simulink model "BS_Adaptive"  (R2018b)
settings: Solver=VariableStepAuto  StartTime=0.0  StopTime=10  RelTol=1e-3
values from neighbouring files (symbols this model uses):
  cond_init = [0, 150/180*pi, pi/3, -pi/2, -3*pi/4,-150/180*pi]'    [init.m]
  hand_des = p(6,:)'    [init.m]
  Law_param = [kd,kd,kd,kd,kd,kd ... (first row only)    [LAUNCH_Backstepping.m]    (also in LAUNCH_Backstepping_Adaptavive.m = [kp,kp,kp,kp,kp,kp; LAUNCH_PD_TRAJ.m = [300000,300000,300000,300000,300000,300000)
  param = param'    [init.m]
  pi_0 = 1    [LAUNCH_Backstepping_Adaptavive.m]
settings Model: Creator=Utente  LastModifiedBy=Utente

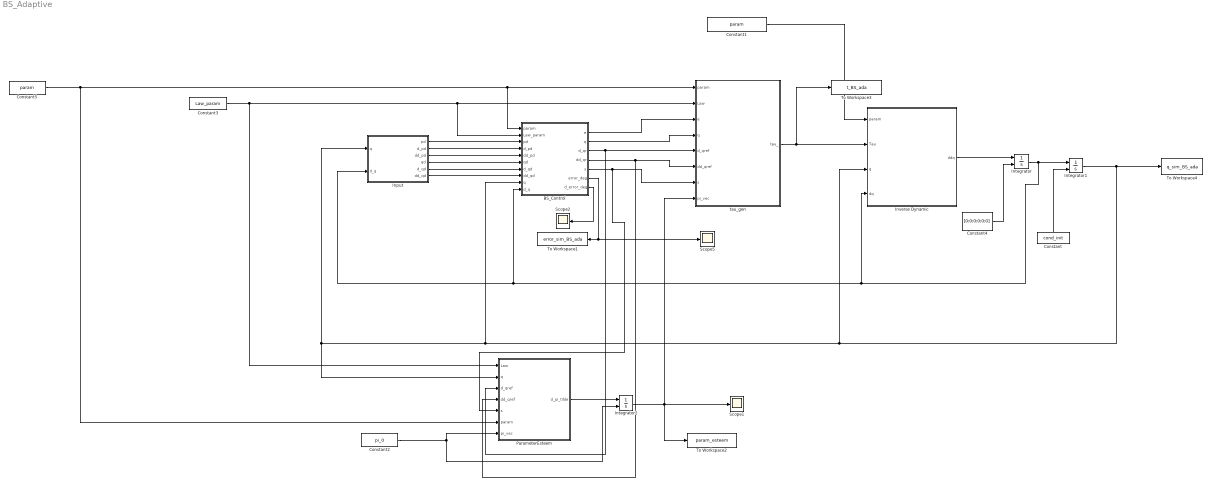
== system BS_Adaptive ==
  BS_Control : MATLAB Function  TreatAsAtomicUnit=on
  Constant : Constant  Value=cond_init
  Constant1 : Constant  Value=param
  Constant2 : Constant  Value=pi_0
  Constant3 : Constant  Value=Law_param
  Constant4 : Constant  Value=[0;0;0;0;0;0]
  Constant5 : Constant  Value=param
  Input : Subsystem
  Integrator : Integrator  InitialConditionSource=external  InitialCondition=[0;0;0;0;0;0]
  Integrator1 : Integrator  InitialConditionSource=external
  Integrator2 : Integrator  InitialConditionSource=external  InitialCondition=[0;0;0;0;0;0]
  Inverse Dynamic : MATLAB Function  TreatAsAtomicUnit=on
  "ParameterEsteem " : MATLAB Function  TreatAsAtomicUnit=on
  Scope1 : Scope
  Scope2 : Scope
  Scope5 : Scope
  To Workspace1 : ToWorkspace  VariableName=error_sim_BS_ada  SaveFormat=Structure With Time  SampleTime=-1
      settings: Save2DSignal=2-D array (concatenate along first dimension)
  To Workspace2 : ToWorkspace  VariableName=param_esteem  SaveFormat=Structure With Time  SampleTime=-1
      settings: Save2DSignal=2-D array (concatenate along first dimension)
  To Workspace3 : ToWorkspace  VariableName=t_BS_ada  SaveFormat=Structure With Time  SampleTime=-1
      settings: Save2DSignal=2-D array (concatenate along first dimension)
  To Workspace4 : ToWorkspace  VariableName=q_sim_BS_ada  SaveFormat=Structure With Time  SampleTime=-1
      settings: Save2DSignal=2-D array (concatenate along first dimension)
  tau_gen : MATLAB Function  TreatAsAtomicUnit=on
  wires:
  Constant1/1 -> Inverse Dynamic/1(param)
  Constant/1 -> Integrator1/2
  Constant4/1 -> Integrator/2
  Inverse Dynamic/1(ddq) -> Integrator/1
  Integrator/1 -> Input/2(d_q), BS_Control/10(d_q), Inverse Dynamic/4(dq), Integrator1/1
  Integrator1/1 -> "ParameterEsteem "/2(q), Input/1(q), BS_Control/9("q "), Inverse Dynamic/3(q), To Workspace4/1
  Constant5/1 -> "ParameterEsteem "/6(param), tau_gen/1(param), BS_Control/1(param)
  Constant3/1 -> "ParameterEsteem "/1(Law), tau_gen/2(Law), BS_Control/2(Law_param)
  Input/6(dd_qd) -> BS_Control/8(dd_qd)
  Input/5(d_qd) -> BS_Control/7(d_qd)
  Input/4(qd) -> BS_Control/6(qd)
  Input/3(dd_pd) -> BS_Control/5(dd_pd)
  Input/2(d_pd) -> BS_Control/4(d_pd)
  Input/1(pd) -> BS_Control/3(pd)
  BS_Control/5(s) -> tau_gen/7(s), "ParameterEsteem "/5(s)
  BS_Control/2(q) -> tau_gen/4(q)
  BS_Control/1(e) -> tau_gen/3(e)
  BS_Control/3(d_qr) -> "ParameterEsteem "/3(d_qref), tau_gen/5(d_qref)
  BS_Control/4(dd_qr) -> "ParameterEsteem "/4(dd_qref), tau_gen/6(dd_qref)
  BS_Control/6(error_deg) -> Scope5/1, To Workspace1/1
  "ParameterEsteem "/1(d_pi_tilde) -> Integrator2/1
  Integrator2/1 -> tau_gen/8(pi_vec), To Workspace2/1, Scope1/1
  Constant2/1 -> Integrator2/2, "ParameterEsteem "/7(pi_vec)
  BS_Control/7(d_error_deg) -> Scope2/1
  tau_gen/1(tau_) -> To Workspace3/1, Inverse Dynamic/2(Tau)

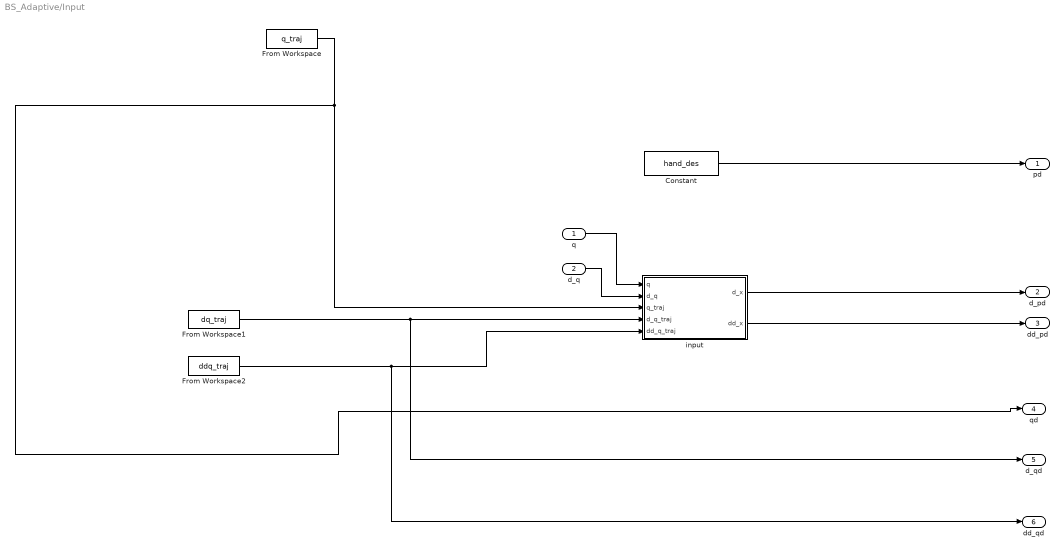
== system BS_Adaptive/Input ==
  q : Inport
  d_q : Inport  Port=2
  Constant : Constant  Value=hand_des
  From Workspace : FromWorkspace  VariableName=q_traj  SampleTime=0
  From Workspace1 : FromWorkspace  VariableName=dq_traj  SampleTime=0
  From Workspace2 : FromWorkspace  VariableName=ddq_traj  SampleTime=0
  "input " : MATLAB Function  TreatAsAtomicUnit=on
  pd : Outport
  d_pd : Outport  Port=2
  dd_pd : Outport  Port=3
  qd : Outport  Port=4
  d_qd : Outport  Port=5
  dd_qd : Outport  Port=6
  wires:
  From Workspace/1 -> "input "/3(q_traj), qd/1
  From Workspace1/1 -> d_qd/1, "input "/4(d_q_traj)
  From Workspace2/1 -> dd_qd/1, "input "/5(dd_q_traj)
  q/1 -> "input "/1(q)
  d_q/1 -> "input "/2(d_q)
  "input "/1(d_x) -> d_pd/1
  "input "/2(dd_x) -> dd_pd/1
  Constant/1 -> pd/1

== matlab function BS_Adaptive/tau_gen ==
  data: param input; Law input; e input; q input; d_qref input; dd_qref input; s input; tau_ output; pi_vec input
function tau_  = tau_gen(param, Law, e, q, d_qref, dd_qref, s, pi_vec)
    
    h = 0.1;
    L7 = 1;
    g = 9.81;

    parameter = [param;
                 L7,h];

    Y = Y_fnu(q,d_qref,dd_qref,parameter,g);
    
    Kd = Law(2)*eye(length(q));
    
    tau_ = Y*[pi_vec(:);1] + Kd*s + e;
    
    
end

== matlab function BS_Adaptive/BS_Control ==
  data: e output; q output; d_qr output; dd_qr output; s output; param input; Law_param input; pd input; d_pd input; dd_pd input; qd input; d_qd input; dd_qd input; q input; d_q input; error_deg output; d_error_deg output
function [e, q , d_qr, dd_qr, s, error_deg, d_error_deg] = BS_Control(param, Law_param, pd, d_pd, dd_pd,qd, d_qd, dd_qd, q, d_q)


    [B,C,G] = Dinamica(param,q,d_q);
    
%     Tau = B*dd_qr + C*d_qr + G + Kd*s + e;

    %SPAZIO OPERATIVO
    Kd = Law_param(1,1)*eye(6);
    L = Law_param(2,1)*eye(6);
    e = qd - q;
    d_e = d_qd - d_q;
    
    d_qr = d_qd + L*e;
    dd_qr = dd_qd + L*d_e;

    s = d_qr - d_q;   
      
    error_deg = e*180/pi;
    d_error_deg = d_e*180/pi;
    
    error_m = e;

    
end

== matlab function BS_Adaptive/Input/input  ==
  data: q input; d_q input; q_traj input; d_x output; d_q_traj input; dd_x output; dd_q_traj input
function [d_x,dd_x] = input_Cond(q, d_q, q_traj, d_q_traj, dd_q_traj)

    JHand = J_hand_fun(q);
    d_JHand = d_Jhand_fun(q,d_q);
    
    d_x = JHand*q_traj;
    dd_x = d_JHand*d_q_traj + JHand*dd_q_traj;
end

== matlab function BS_Adaptive/Inverse Dynamic ==
  data: param input; Tau input; ddq output; q input; dq input
function ddq = inverseD(param,Tau,q,dq)

    [B,C,G] = Dinamica(param,q,dq);
    tot = Tau - C*dq - G;
    
    ddq = B\(tot);
    
end

== matlab function BS_Adaptive/ParameterEsteem  ==
  data: Law input; q input; d_qref input; dd_qref input; s input; param input; d_pi_tilde output; pi_vec input
function d_pi_tilde = ParamEsteem(Law, q, d_qref, dd_qref, s, param, pi_vec)
    
    R = Law(3,1)*eye(size([pi_vec;1]));
    h = 0.1;
    L7 = 1;
    g = 9.81;

    parameter = [param;
                 L7,h];

    Y = Y_fnu(q,d_qref,dd_qref,parameter,g);
    
    d_pi_tilde = R\Y'*s;
    
end
